simulink model "QPProblem"  (R2021a)
settings: Solver=ode4  StartTime=0.0  StopTime=0.1  FixedStep=0.1  RelTol=1e-3
settings Model: Creator=isak.skeie  LastModifiedBy=isak.skeie

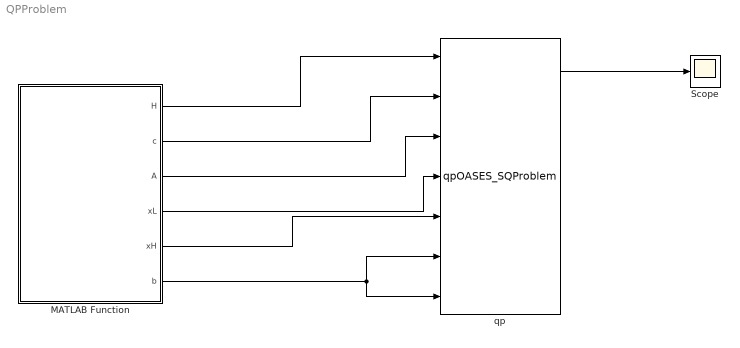
== system QPProblem ==
  MATLAB Function : MATLAB Function  TreatAsAtomicUnit=on
  Scope : Scope
  qp : S-Function  FunctionName=qpOASES_SQProblem  SFunctionDeploymentMode=off  EnableBusSupport=off
  wires:
  MATLAB Function/1(H) -> qp/1
  MATLAB Function/2(c) -> qp/2
  MATLAB Function/3(A) -> qp/3
  MATLAB Function/4(xL) -> qp/4
  MATLAB Function/5(xH) -> qp/5
  MATLAB Function/6(b) -> qp/7, qp/6
  qp/1 -> Scope/1

== matlab function QPProblem/MATLAB Function ==
  data: H output; c output; A output; xL output; xH output; b output
function [H, c, A, xL, xH, b] = QR_Problem()




%Make matrices and vectors



%Hessian matric H
H_mat = diag([6,0,-10]);

    %Need to stack elements in matrix column wise for solver
    H = H_mat(:);


%C Matrix
%Linear Term vector
c = [2.5 7 0]';


%A matrix
%Equality constraints

A_mat = [2 3 4;
         -3 0 -8;
         -4 -3.2 1.8];
A = A_mat(:);


%RHX of equality constraints
b = [5 -6 2]';

%Bounds
xL = [-inf -inf -inf]';
xH = [inf inf inf]';
